simulink model "sweepsine"  (R2018b)
settings: Solver=FixedStepAuto  StartTime=0.0  StopTime=20  FixedStep=0.001  RelTol=1e-3
settings Model: Creator=lubuntu  LastModifiedBy=lubuntu

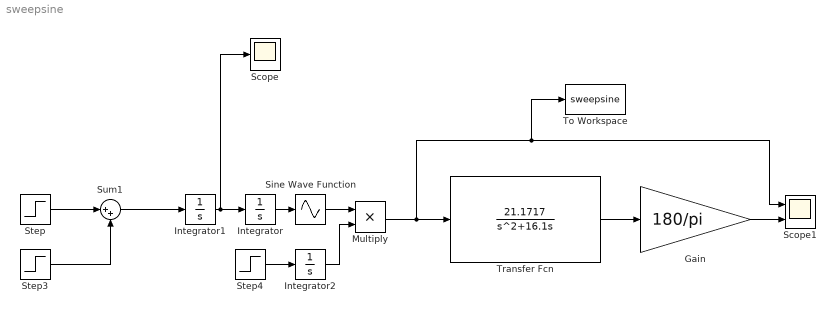
== system sweepsine ==
  Gain : Gain  Gain=180/pi
  Integrator : Integrator
  Integrator1 : Integrator
  Integrator2 : Integrator  LimitOutput=on  UpperSaturationLimit=7  LowerSaturationLimit=0
  Multiply : Product
  Scope : Scope
  Scope1 : Scope  NumInputPorts=2
  Sine Wave Function : Sin  TimeSource=Use external signal  SampleTime=0
  Step : Step  After=100  SampleTime=0
  Step3 : Step  Time=1.05  After=-99  SampleTime=0
  Step4 : Step  SampleTime=0
  Sum1 : Sum  Inputs=|++
  To Workspace : ToWorkspace  VariableName=sweepsine  SaveFormat=Timeseries  SampleTime=-1
  Transfer Fcn : TransferFcn  Numerator=[ 21.1717 ]  Denominator=[1 16.1 0]
  wires:
  Integrator/1 -> Sine Wave Function/1
  Transfer Fcn/1 -> Gain/1
  Multiply/1 -> Transfer Fcn/1, To Workspace/1, Scope1/1
  Sine Wave Function/1 -> Multiply/1
  Step/1 -> Sum1/1
  Sum1/1 -> Integrator1/1
  Integrator1/1 -> Scope/1, Integrator/1
  Gain/1 -> Scope1/2
  Integrator2/1 -> Multiply/2
  Step4/1 -> Integrator2/1
  Step3/1 -> Sum1/2
